simulink subsystem "Servo_motor"  (R2020a)
settings: Solver=VariableStepAuto  StartTime=0.0  StopTime=10.0  RelTol=1e-3
values from neighbouring files (symbols this model uses):
  Eref = 5    [Servo_motor.mat]
settings Model: Creator=Haier  LastModifiedBy=Haier

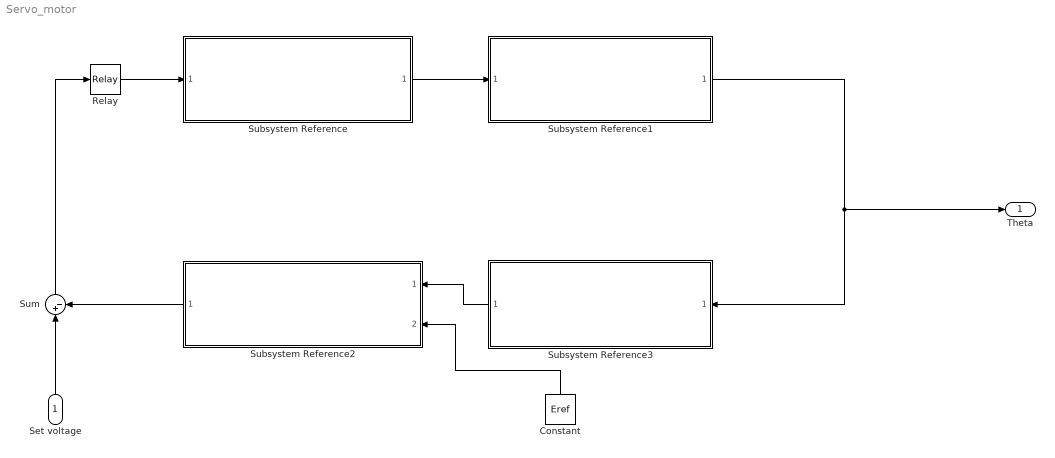
== system Servo_motor ==
  Set voltage : Inport
  Constant : Constant  Value=Eref
  Relay : Relay  OnOutputValue=5
  Subsystem Reference : Subsystem  ReferencedSubsystem=Motor_subsystem
  Subsystem Reference1 : Subsystem  ReferencedSubsystem=Gearbox1
  Subsystem Reference2 : Subsystem  ReferencedSubsystem=Rotary_Encoder
  Subsystem Reference3 : Subsystem  ReferencedSubsystem=Gearbox1
  Sum : Sum  Inputs=|+-
  Theta : Outport
  wires:
  Subsystem Reference/1 -> Subsystem Reference1/1
  Subsystem Reference3/1 -> Subsystem Reference2/1
  Subsystem Reference1/1 -> Subsystem Reference3/1, Theta/1
  Constant/1 -> Subsystem Reference2/2
  Set voltage/1 -> Sum/1
  Subsystem Reference2/1 -> Sum/2
  Sum/1 -> Relay/1
  Relay/1 -> Subsystem Reference/1
